simulink model "TestBench__Buffer_Block"  (R2023b)
settings: Solver=FixedStepDiscrete  StartTime=0.0  StopTime=0.5  FixedStep=1/600  RelTol=1e-3
libraries: dspsigops x1, matrix_library x1
settings Model: Creator=leoni  LastModifiedBy=leoni

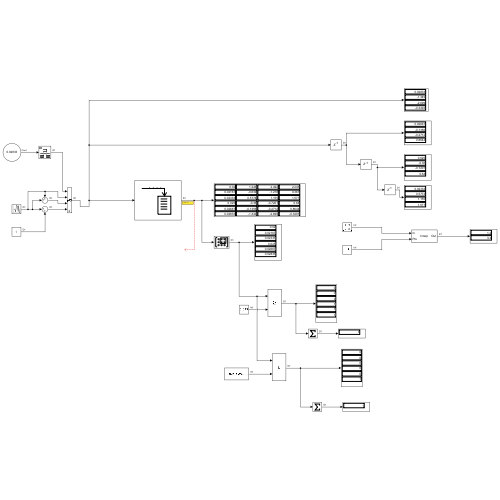
[thumbnail: Simulink's stored preview of the top-level diagram]
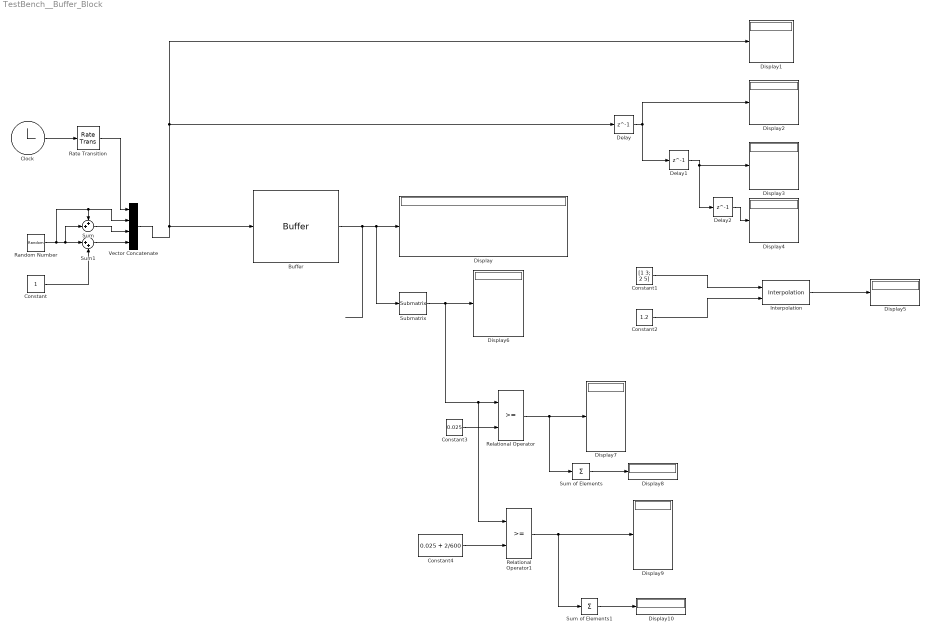
== system TestBench__Buffer_Block ==
  Buffer : Buffer  N=6  V=5  OutputFrames=off
  Clock : Clock
      settings: Decimation=3
  Constant : Constant  SampleTime=-1
  Constant1 : Constant  Value=[1 3; 2 5]
  Constant2 : Constant  Value=1.2
  Constant3 : Constant  Value=0.025
  Constant4 : Constant  Value=0.025 + 2/600
  Delay : Delay  DelayLength=1
  Delay1 : Delay  DelayLength=1
  Delay2 : Delay  DelayLength=1
  Display{,1..10} (11 alike) : Display
  Interpolation : dspsigops/Interpolation  InterpSource=Input port  InterpPoints=[1.1 4.8 2.67 1.6 3.2]'  InterpMode=Linear  InterpL=3  InterpR=3  InterpAlpha=0.5  InvalidMode=Error
  Random Number : RandomNumber  SampleTime=1/600
  Rate Transition : RateTransition
  Relational Operator : RelationalOperator  OutDataTypeStr=boolean  RndMeth=Simplest  InputSameDT=off
  Relational Operator1 : RelationalOperator  OutDataTypeStr=boolean  RndMeth=Simplest  InputSameDT=off
  Submatrix : matrix_library/Submatrix  RowSpan=All rows  RowStartMode=First  RowStartIndex=1  RowEndMode=Last  RowEndIndex=1  ColSpan=One column  ColStartMode=First  ColStartIndex=1  ColEndMode=Last  ColEndIndex=1
  Sum : Sum  Inputs=++|
  Sum of Elements : Sum  Inputs=+
  Sum of Elements1 : Sum  Inputs=+
  Sum1 : Sum  Inputs=|++
  Vector Concatenate : Concatenate  NumInputs=4  Mode=Multidimensional array  ConcatenateDimension=2
  wires:
  Random Number/1 -> Vector Concatenate/2, Sum/1, Sum1/1, Sum/2
  Sum/1 -> Vector Concatenate/3
  Sum1/1 -> Vector Concatenate/4
  Constant/1 -> Sum1/2
  Buffer/1 -> Submatrix/1, Display/1
  Delay/1 -> Delay1/1, Display2/1
  Delay1/1 -> Delay2/1, Display3/1
  Delay2/1 -> Display4/1
  Clock/1 -> Rate Transition/1
  Rate Transition/1 -> Vector Concatenate/1
  Vector Concatenate/1 -> Buffer/1, Delay/1, Display1/1
  Constant2/1 -> Interpolation/2
  Constant1/1 -> Interpolation/1
  Interpolation/1 -> Display5/1
  Submatrix/1 -> Relational Operator1/1, Relational Operator/1, Display6/1
  Constant3/1 -> Relational Operator/2
  Relational Operator/1 -> Sum of Elements/1, Display7/1
  Sum of Elements/1 -> Display8/1
  Constant4/1 -> Relational Operator1/2
  Sum of Elements1/1 -> Display10/1
  Relational Operator1/1 -> Sum of Elements1/1, Display9/1
